simulink subsystem "AS5600_Sensor"  (R2022b)
settings: Solver=VariableStepAuto  StartTime=0.0  StopTime=10.0  RelTol=1e-3
model mask{delta_th=0.5, wrap=on}
  mask prompts: delta_th "Angle quantization step:"; wrap "Wrap angle:"
settings Model: Creator=gotta  LastModifiedBy=gotta

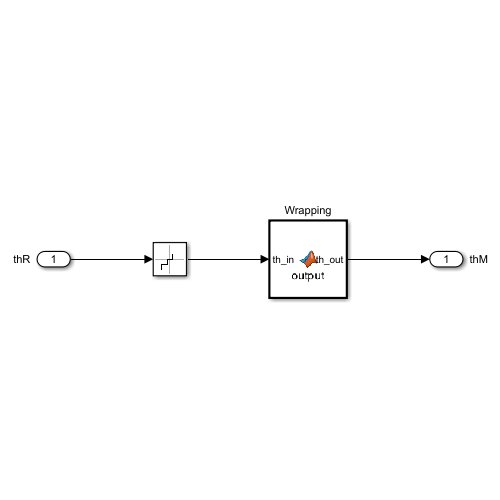
[thumbnail: Simulink's stored preview of the top-level diagram]
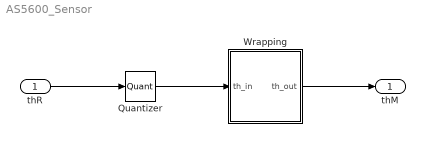
== system AS5600_Sensor ==
  thR : Inport
  Quantizer : Quantizer  QuantizationInterval=delta_th  SampleTime=1e-3
  Wrapping : MATLAB Function  TreatAsAtomicUnit=on
  thM : Outport
  wires:
  thR/1 -> Quantizer/1
  Wrapping/1(th_out) -> thM/1
  Quantizer/1 -> Wrapping/1(th_in)

== matlab function AS5600_Sensor/Wrapping ==
  data: th_in input; th_out output; wrap parameter
function th_out = output(th_in, wrap)

% wrapping angle
if wrap == 1
    th_out = wrapTo2Pi(th_in);
else
    th_out = th_in;
end
